simulink model "acquisition"  (R2020a)
settings: Solver=VariableStepAuto  StartTime=0.0  StopTime=simulation_time  RelTol=1e-3
values from neighbouring files (symbols this model uses):
  ca_fft_coef = zeros(37,4096)    [acquisition_hw_init.m]
  ca_fft_width = 14    [acquisition_hw_init.m]
  core_upsample_ratio = 24    [acquisition_hw_init.m]
  correlator_latency = 19    [acquisition_hw_init.m]
  ddc_latency = 5    [acquisition_hw_init.m]
  DDS_signal_width = 12    [acquisition_hw_init.m]
  f_start_phase = core_upsample_ratio*f_start/fs    (= -0.0006103515625)    [acquisition_hw_init.m]
  fd_phase_increment = core_upsample_ratio*(f_dds_change)/fs    (= 2e-05)    [acquisition_hw_init.m]
  fft_length = 4096    [acquisition_hw_init.m]
  fs = core_upsample_ratio*fs_adc    (= 120000000)    [acquisition_hw_init.m]
  ts = 1/fs    [acquisition_debugger_data.m]    (also in acquisition_hw_init.m = 8.33333333333e-09)
  ts_adc = 1/fs_adc    (= 2e-07)    [acquisition_hw_init.m]
libraries: xbsIndex_r4 x325
(part 1 of 2)
settings Model: Creator=NoiseIran  LastModifiedBy=sysgen

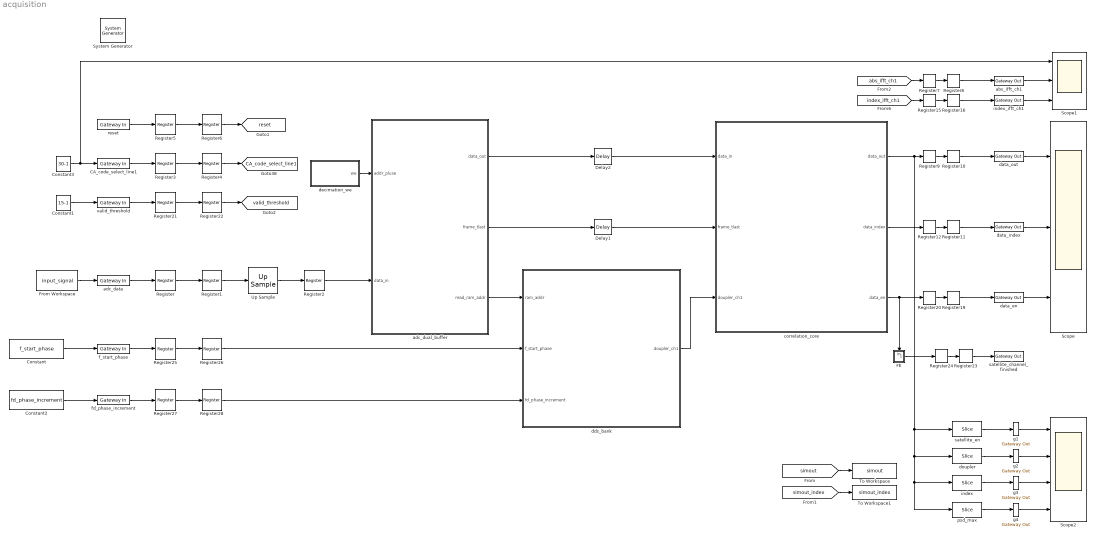
== system acquisition ==
  " System Generator" : xbsIndex_r4/ System Generator  Tag=genX  xilinxfamily=zynq  part=xc7z020  speed=-1  package=clg400  synthesis_tool=Vivado  clock_wrapper=Clock Enables  directory=./netlist  proj_type=Vivado  Synth_file=Vivado Synthesis Defaults  Impl_file=Vivado Implementation Defaults  testbench=off  simulink_period=ts  sysclk_period=ts*1e9  dcm_input_clock_period=10  incr_netlist=off  trim_vbits=Everywhere in SubSystem  dbl_ovrd=According to Block Masks  core_generation=According to Block Masks  run_coregen=off  deprecated_control=off  eval_field=0  block_type=sysgen
  CA_code_select_line1 : xbsIndex_r4/Gateway In  gui_display_data_type=Fixed-point  arith_type=Unsigned  n_bits=6  bin_pt=0  preci_type=Single  exp_width=8  frac_width=24  rows=1  columns=1  quantization="Round  (unbiased: +/- Inf)"  overflow=Saturate  period=ts  UseAsADC=off  ADCChannel='1'  interface=None  automatic_assignment=on  address_offset=hex2dec('00')  intf_name=''  intf_description=''  default_value=0  timing_constraint=None  locs_specified=off  LOCs={}  io_standard={}  inherit_from_input=off  hdl_port=on  dbl_ovrd=off  block_type=gatewayin
  Constant : Constant  Value=f_start_phase
  Constant1 : Constant  Value=15-1
  Constant2 : Constant  Value=fd_phase_increment
  Constant3 : Constant  Value=30-1
  Delay1 : xbsIndex_r4/Delay  rst=off  infoeditControl=Selection of Reset will increase slice count due to use of real FFs and instead of SRLs  en=off  latency=ddc_latency  reg_retiming=off  dbl_ovrd=off  block_type=delay
  Delay2 : xbsIndex_r4/Delay  rst=off  infoeditControl=Selection of Reset will increase slice count due to use of real FFs and instead of SRLs  en=off  latency=ddc_latency  reg_retiming=off  dbl_ovrd=off  block_type=delay
  FE : Subsystem
      settings: PortSchema="{\"entries\":[{\"content\":{\"sides\":[{\"content\":{\"connectorIds\":[]},\"type\":\"ConnectorPlacement.EquallySpacedRectSide\",\"uuid\":\"2043c5b6-9866-4807-b8e4-2bcf4a8da4e0\"},{\"content\":{\"connectorIds\":[\"Out1\"],\"side\":\"RIGHT\"},\"type\":\"ConnectorPlacement.EquallySpacedRectSide\",\"uuid\":\"05fb68c1-bf14-4cfd-8c41-78b1f158a67a\"},{\"content\":{\"connectorIds\":[\"In1\"],\"side\":\"TOP\"},\"type\":\"ConnectorPlacement.EquallySpacedRectSide\",\"uuid\":\"9a584094-bda8-44b5-9f18-145d2f87f2be\"}]},\"type\":\"ConnectorPlacement.EquallySpacedConnector\",\"uuid\":\"61bf9f6d-0cb1-4913-8ccd-914b8e14feb8\"}],\"packageUris\":[\"http://schema.mathworks.com/mf0/Connector/19700101\"],\"version\":\"1.0\"}"
  From Workspace : FromWorkspace  VariableName=input_signal  SampleTime=ts_adc
  Register{,1..4,7..12,15..16,19..28} (23 alike) : xbsIndex_r4/Register  init=0  rst=off  en=off  dbl_ovrd=off  block_type=register
  Register5 : xbsIndex_r4/Register  init=1  rst=off  en=off  dbl_ovrd=off  block_type=register
  Register6 : xbsIndex_r4/Register  init=1  rst=off  en=off  dbl_ovrd=off  block_type=register
  Scope : Scope  NumInputPorts=3
  Scope1 : Scope  NumInputPorts=3
  Scope2 : Scope  NumInputPorts=4
  To Workspace : ToWorkspace  VariableName=simout  SaveFormat=Structure With Time  SampleTime=-1
  To Workspace1 : ToWorkspace  VariableName=simout_index  SaveFormat=Structure With Time  SampleTime=-1
  Up Sample : xbsIndex_r4/Up Sample  sample_ratio=core_upsample_ratio  copy_samples=on  en=off  latency=1  dbl_ovrd=off  block_type=usamp
  abs_ifft_ch1 : xbsIndex_r4/Gateway Out  inherit_from_input=off  hdl_port=on  rows=1  columns=1  UseAsDAC=off  DACChannel='1'  interface=None  automatic_assignment=on  address_offset=hex2dec('00')  intf_name=''  intf_description=''  timing_constraint=None  locs_specified=off  LOCs={}  io_standard={}  block_type=gatewayout
  adc_data : xbsIndex_r4/Gateway In  gui_display_data_type=Fixed-point  arith_type="Signed  (2's comp)"  n_bits=input_signal_width  bin_pt=input_signal_binary_point  preci_type=Single  exp_width=8  frac_width=24  rows=1  columns=1  quantization="Round  (unbiased: +/- Inf)"  overflow=Saturate  period=ts_adc  UseAsADC=off  ADCChannel='1'  interface=None  automatic_assignment=on  address_offset=hex2dec('00')  intf_name=''  intf_description=''  default_value=0  timing_constraint=None  locs_specified=off  LOCs={}  io_standard={}  inherit_from_input=off  hdl_port=on  dbl_ovrd=off  block_type=gatewayin
  adc_dual_buffer : Subsystem
  correlation_core : Subsystem
  data_en : xbsIndex_r4/Gateway Out  inherit_from_input=off  hdl_port=on  rows=1  columns=1  UseAsDAC=off  DACChannel='1'  interface=None  automatic_assignment=on  address_offset=hex2dec('00')  intf_name=''  intf_description=''  timing_constraint=None  locs_specified=off  LOCs={}  io_standard={}  block_type=gatewayout
  data_index : xbsIndex_r4/Gateway Out  inherit_from_input=off  hdl_port=on  rows=1  columns=1  UseAsDAC=off  DACChannel='1'  interface=None  automatic_assignment=on  address_offset=hex2dec('00')  intf_name=''  intf_description=''  timing_constraint=None  locs_specified=off  LOCs={}  io_standard={}  block_type=gatewayout
  data_out : xbsIndex_r4/Gateway Out  inherit_from_input=off  hdl_port=on  rows=1  columns=1  UseAsDAC=off  DACChannel='1'  interface=None  automatic_assignment=on  address_offset=hex2dec('00')  intf_name=''  intf_description=''  timing_constraint=None  locs_specified=off  LOCs={}  io_standard={}  block_type=gatewayout
  dds_bank : Subsystem
  decimation_we : Subsystem
  doupler : xbsIndex_r4/Slice  nbits=24  boolean_output=off  mode=Lower Bit Location + Width  bit1=0  base1=MSB of Input  bit0=20  base0=LSB of Input  dbl_ovrd=off  block_type=slice
  f_start_phase : xbsIndex_r4/Gateway In  gui_display_data_type=Fixed-point  arith_type="Signed  (2's comp)"  n_bits=DDS_phase_width  bin_pt=DDS_phase_width  preci_type=Single  exp_width=8  frac_width=24  rows=1  columns=1  quantization="Round  (unbiased: +/- Inf)"  overflow=Saturate  period=ts  UseAsADC=off  ADCChannel='1'  interface=None  automatic_assignment=on  address_offset=hex2dec('00')  intf_name=''  intf_description=''  default_value=0  timing_constraint=None  locs_specified=off  LOCs={}  io_standard={}  inherit_from_input=off  hdl_port=on  dbl_ovrd=off  block_type=gatewayin
  fd_phase_increment : xbsIndex_r4/Gateway In  gui_display_data_type=Fixed-point  arith_type="Signed  (2's comp)"  n_bits=DDS_phase_width  bin_pt=DDS_phase_width  preci_type=Single  exp_width=8  frac_width=24  rows=1  columns=1  quantization="Round  (unbiased: +/- Inf)"  overflow=Saturate  period=ts  UseAsADC=off  ADCChannel='1'  interface=None  automatic_assignment=on  address_offset=hex2dec('00')  intf_name=''  intf_description=''  default_value=0  timing_constraint=None  locs_specified=off  LOCs={}  io_standard={}  inherit_from_input=off  hdl_port=on  dbl_ovrd=off  block_type=gatewayin
  g{1..4} (4 alike) : xbsIndex_r4/Gateway Out  inherit_from_input=off  hdl_port=off  rows=1  columns=1  UseAsDAC=off  DACChannel='1'  interface=None  automatic_assignment=on  address_offset=hex2dec('00')  intf_name=''  intf_description=''  timing_constraint=None  locs_specified=off  LOCs={}  io_standard={}  block_type=gatewayout
  index : xbsIndex_r4/Slice  nbits=12  boolean_output=off  mode=Lower Bit Location + Width  bit1=0  base1=MSB of Input  bit0=8  base0=LSB of Input  dbl_ovrd=off  block_type=slice
  index_ifft_ch1 : xbsIndex_r4/Gateway Out  inherit_from_input=off  hdl_port=on  rows=1  columns=1  UseAsDAC=off  DACChannel='1'  interface=None  automatic_assignment=on  address_offset=hex2dec('00')  intf_name=''  intf_description=''  timing_constraint=None  locs_specified=off  LOCs={}  io_standard={}  block_type=gatewayout
  psd_max : xbsIndex_r4/Slice  nbits=8  boolean_output=off  mode=Lower Bit Location + Width  bit1=0  base1=MSB of Input  bit0=0  base0=LSB of Input  dbl_ovrd=off  block_type=slice
  reset : xbsIndex_r4/Gateway In  gui_display_data_type=Boolean  arith_type=Boolean  n_bits=4  bin_pt=0  preci_type=Single  exp_width=8  frac_width=24  rows=1  columns=1  quantization="Round  (unbiased: +/- Inf)"  overflow=Saturate  period=ts  UseAsADC=off  ADCChannel='1'  interface=None  automatic_assignment=on  address_offset=hex2dec('00')  intf_name=''  intf_description=''  default_value=0  timing_constraint=None  locs_specified=off  LOCs={}  io_standard={}  inherit_from_input=off  hdl_port=on  dbl_ovrd=off  block_type=gatewayin
  satellite_channel_finished : xbsIndex_r4/Gateway Out  inherit_from_input=off  hdl_port=on  rows=1  columns=1  UseAsDAC=off  DACChannel='1'  interface=None  automatic_assignment=on  address_offset=hex2dec('00')  intf_name=''  intf_description=''  timing_constraint=None  locs_specified=off  LOCs={}  io_standard={}  block_type=gatewayout
  satellite_en : xbsIndex_r4/Slice  nbits=1  boolean_output=on  mode=Lower Bit Location + Width  bit1=0  base1=MSB of Input  bit0=44  base0=LSB of Input  dbl_ovrd=off  block_type=slice
  valid_threshold : xbsIndex_r4/Gateway In  gui_display_data_type=Fixed-point  arith_type="Signed  (2's comp)"  n_bits=abs_adder_width  bin_pt=abs_adder_point  preci_type=Single  exp_width=8  frac_width=24  rows=1  columns=1  quantization="Round  (unbiased: +/- Inf)"  overflow=Saturate  period=ts  UseAsADC=off  ADCChannel='1'  interface=None  automatic_assignment=on  address_offset=hex2dec('00')  intf_name=''  intf_description=''  default_value=0  timing_constraint=None  locs_specified=off  LOCs={}  io_standard={}  inherit_from_input=off  hdl_port=on  dbl_ovrd=off  block_type=gatewayin
  tag scope: CA_code_select_line1=global, reset=global, valid_threshold=global
  wires:
  Register/1 -> Register1/1
  adc_data/1 -> Register/1
  Register1/1 -> Up Sample/1
  Up Sample/1 -> Register2/1
  Register2/1 -> adc_dual_buffer/2(data_in)
  adc_dual_buffer/3(read_ram_addr) -> dds_bank/1(ram_addr)
  From Workspace/1 -> adc_data/1
  adc_dual_buffer/1(data_out) -> Delay2/1
  CA_code_select_line1/1 -> Register3/1
  Register3/1 -> Register4/1
  Register4/1 -> [CA_code_select_line1]
  reset/1 -> Register5/1
  Register5/1 -> Register6/1
  Register6/1 -> [reset]
  decimation_we/1(we) -> adc_dual_buffer/1(addr_pluse)
  Register8/1 -> abs_ifft_ch1/1
  Register7/1 -> Register8/1
  dds_bank/1(doupler_ch1) -> correlation_core/3(doupler_ch1)
  [abs_ifft_ch1] -> Register7/1
  Register16/1 -> index_ifft_ch1/1
  Register15/1 -> Register16/1
  [index_ifft_ch1] -> Register15/1
  correlation_core/1(data_out) -> psd_max/1, index/1, doupler/1, satellite_en/1, Register9/1
  Register9/1 -> Register10/1
  Register11/1 -> data_index/1
  Register12/1 -> Register11/1
  correlation_core/2(data_index) -> Register12/1
  Register20/1 -> Register19/1
  Register19/1 -> data_en/1
  correlation_core/3(data_en) -> FE/1(in), Register20/1
  data_out/1 -> Scope/1
  data_index/1 -> Scope/2
  data_en/1 -> Scope/3
  abs_ifft_ch1/1 -> Scope1/2
  index_ifft_ch1/1 -> Scope1/3
  Register21/1 -> Register22/1
  valid_threshold/1 -> Register21/1
  Register22/1 -> [valid_threshold]
  Constant1/1 -> valid_threshold/1
  Register24/1 -> Register23/1
  Register23/1 -> satellite_channel_finished/1
  FE/1(fe) -> Register24/1
  Register10/1 -> data_out/1
  satellite_en/1 -> g1/1
  doupler/1 -> g2/1
  index/1 -> g3/1
  psd_max/1 -> g4/1
  Constant2/1 -> fd_phase_increment/1
  Constant/1 -> f_start_phase/1
  f_start_phase/1 -> Register25/1
  fd_phase_increment/1 -> Register27/1
  Register25/1 -> Register26/1
  Register26/1 -> dds_bank/2(f_start_phase)
  Register27/1 -> Register28/1
  Register28/1 -> dds_bank/3(fd_phase_increment)
  adc_dual_buffer/2(frame_tlast) -> Delay1/1
  Delay2/1 -> correlation_core/1(data_in)
  Delay1/1 -> correlation_core/2(frame_tlast)
  [simout] -> To Workspace/1
  [simout_index] -> To Workspace1/1
  Constant3/1 -> Scope1/1, CA_code_select_line1/1
  g1/1 -> Scope2/1
  g2/1 -> Scope2/2
  g3/1 -> Scope2/3
  g4/1 -> Scope2/4

== system acquisition/FE ==
  in : Inport
  Delay : xbsIndex_r4/Delay  rst=off  infoeditControl=Selection of Reset will increase slice count due to use of real FFs and instead of SRLs  en=off  latency=1  reg_retiming=off  dbl_ovrd=off  block_type=delay
  Inverter : xbsIndex_r4/Inverter  en=off  latency=0  dbl_ovrd=off  block_type=inv
  Logical : xbsIndex_r4/Logical  logical_function=AND  inputs=2  en=off  latency=0  precision=Full  arith_type=Unsigned  n_bits=16  bin_pt=0  align_bp=on  dbl_ovrd=off  block_type=logical
  fe : Outport
  wires:
  in/1 -> Inverter/1, Delay/1
  Inverter/1 -> Logical/1
  Delay/1 -> Logical/2
  Logical/1 -> fe/1

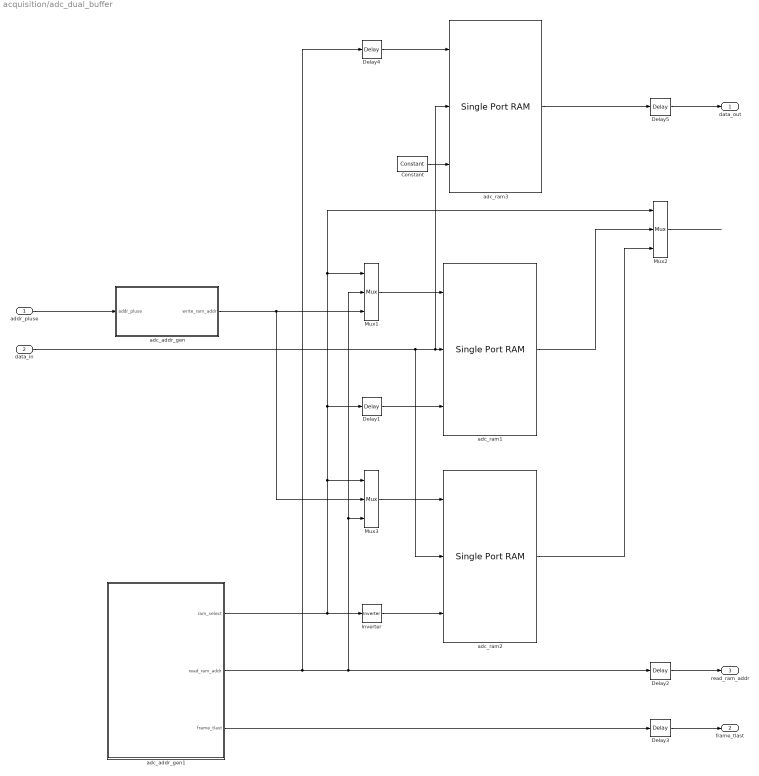
== system acquisition/adc_dual_buffer ==
  addr_pluse : Inport
  data_in : Inport  Port=2
  Constant : xbsIndex_r4/Constant  const=0  gui_display_data_type=Boolean  arith_type=Boolean  n_bits=16  bin_pt=14  preci_type=Single  exp_width=8  frac_width=24  explicit_period=on  period=ts  equ=P=C  opselect=C  inp2=PCIN>>17  opr=+  inp1=P  carry=CIN  dbl_ovrd=off  block_type=constant
  Delay1 : xbsIndex_r4/Delay  rst=off  infoeditControl=Selection of Reset will increase slice count due to use of real FFs and instead of SRLs  en=off  latency=1  reg_retiming=off  dbl_ovrd=off  block_type=delay
  Delay2 : xbsIndex_r4/Delay  rst=off  infoeditControl=Selection of Reset will increase slice count due to use of real FFs and instead of SRLs  en=off  latency=adc_addr_gen_latency  reg_retiming=off  dbl_ovrd=off  block_type=delay
  Delay3 : xbsIndex_r4/Delay  rst=off  infoeditControl=Selection of Reset will increase slice count due to use of real FFs and instead of SRLs  en=off  latency=adc_addr_gen_latency  reg_retiming=off  dbl_ovrd=off  block_type=delay
  Delay4 : xbsIndex_r4/Delay  rst=off  infoeditControl=Selection of Reset will increase slice count due to use of real FFs and instead of SRLs  en=off  latency=1  reg_retiming=off  dbl_ovrd=off  block_type=delay
  Delay5 : xbsIndex_r4/Delay  rst=off  infoeditControl=Selection of Reset will increase slice count due to use of real FFs and instead of SRLs  en=off  latency=1  reg_retiming=off  dbl_ovrd=off  block_type=delay
  Inverter : xbsIndex_r4/Inverter  en=off  latency=1  dbl_ovrd=off  block_type=inv
  Mux1 : xbsIndex_r4/Mux  inputs=2  en=off  latency=1  precision=Full  arith_type=Unsigned  n_bits=16  bin_pt=14  quantization=Truncate  overflow=Wrap  dbl_ovrd=off  block_type=mux
  Mux2 : xbsIndex_r4/Mux  inputs=2  en=off  latency=1  precision=Full  arith_type=Unsigned  n_bits=16  bin_pt=14  quantization=Truncate  overflow=Wrap  dbl_ovrd=off  block_type=mux
  Mux3 : xbsIndex_r4/Mux  inputs=2  en=off  latency=1  precision=Full  arith_type=Unsigned  n_bits=16  bin_pt=14  quantization=Truncate  overflow=Wrap  dbl_ovrd=off  block_type=mux
  adc_addr_gen : Subsystem
  adc_addr_gen1 : Subsystem
  adc_ram1 : xbsIndex_r4/Single Port RAM  depth=fft_length  initVector=adc_ram_init  distributed_mem=Block RAM  write_mode=Read After Write  rst=off  init_reg=0  en=off  optimize_latency=off  latency=1  optimize=Speed  dbl_ovrd=off  simulation_type=fast_sim  block_type=spram
  adc_ram2 : xbsIndex_r4/Single Port RAM  depth=fft_length  initVector=adc_ram_init  distributed_mem=Block RAM  write_mode=Read After Write  rst=off  init_reg=0  en=off  optimize_latency=off  latency=1  optimize=Speed  dbl_ovrd=off  simulation_type=fast_sim  block_type=spram
  adc_ram3 : xbsIndex_r4/Single Port RAM  depth=fft_length  initVector=adc_ram_init  distributed_mem=Block RAM  write_mode=Read After Write  rst=off  init_reg=0  en=off  optimize_latency=off  latency=1  optimize=Speed  dbl_ovrd=off  simulation_type=fast_sim  block_type=spram
  data_out : Outport
  frame_tlast : Outport  Port=2
  read_ram_addr : Outport  Port=3
  wires:
  Mux1/1 -> adc_ram1/1
  Inverter/1 -> adc_ram2/3
  Mux3/1 -> adc_ram2/1
  adc_addr_gen/1(write_ram_addr) -> Mux3/2, Mux1/3
  adc_addr_gen1/1(ram_select) -> Mux2/1, Mux1/1, Delay1/1, Mux3/1, Inverter/1
  adc_ram1/1 -> Mux2/2
  adc_ram2/1 -> Mux2/3
  Delay1/1 -> adc_ram1/3
  addr_pluse/1 -> adc_addr_gen/1(addr_pluse)
  Mux2/1 -> ?
  Delay2/1 -> read_ram_addr/1
  adc_addr_gen1/3(frame_tlast) -> Delay3/1
  Delay3/1 -> frame_tlast/1
  adc_addr_gen1/2(read_ram_addr) -> Delay4/1, Mux1/2, Mux3/3, Delay2/1
  data_in/1 -> adc_ram3/2, adc_ram1/2, adc_ram2/2
  Constant/1 -> adc_ram3/3
  Delay4/1 -> adc_ram3/1
  adc_ram3/1 -> Delay5/1
  Delay5/1 -> data_out/1

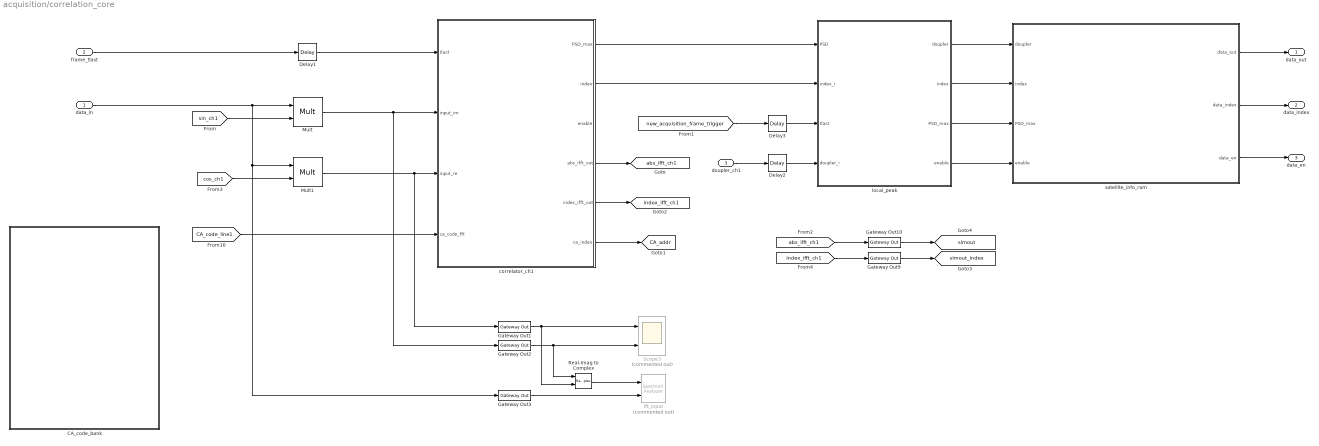
== system acquisition/correlation_core ==
  data_in : Inport
  frame_tlast : Inport  Port=2
  doupler_ch1 : Inport  Port=3
  CA_code_bank : Subsystem
  Delay1 : xbsIndex_r4/Delay  rst=off  infoeditControl=Selection of Reset will increase slice count due to use of real FFs and instead of SRLs  en=off  latency=3  reg_retiming=off  dbl_ovrd=off  block_type=delay
  Delay2 : xbsIndex_r4/Delay  rst=off  infoeditControl=Selection of Reset will increase slice count due to use of real FFs and instead of SRLs  en=off  latency=correlator_latency  reg_retiming=off  dbl_ovrd=off  block_type=delay
  Delay3 : xbsIndex_r4/Delay  rst=off  infoeditControl=Selection of Reset will increase slice count due to use of real FFs and instead of SRLs  en=off  latency=correlator_latency+ddc_latency  reg_retiming=off  dbl_ovrd=off  block_type=delay
  Gateway Out{1..3,9..10} (5 alike) : xbsIndex_r4/Gateway Out  inherit_from_input=off  hdl_port=off  rows=1  columns=1  UseAsDAC=off  DACChannel='1'  interface=None  automatic_assignment=on  address_offset=hex2dec('00')  intf_name=''  intf_description=''  timing_constraint=None  locs_specified=off  LOCs={}  io_standard={}  block_type=gatewayout
  Mult : xbsIndex_r4/Mult  precision=User Defined  arith_type="Signed  (2's comp)"  n_bits=multiplier_width  bin_pt=multiplier_point  quantization="Round  (unbiased: +/- Inf)"  overflow=Saturate  en=off  latency=3  use_behavioral_HDL=off  opt=Speed  use_embedded=on  optimum_pipeline=off  pipeline=on  dbl_ovrd=off  use_rpm=on  placement_style=Triangular  block_type=mult
  Mult1 : xbsIndex_r4/Mult  precision=User Defined  arith_type="Signed  (2's comp)"  n_bits=multiplier_width  bin_pt=multiplier_point  quantization="Round  (unbiased: +/- Inf)"  overflow=Saturate  en=off  latency=3  use_behavioral_HDL=off  opt=Speed  use_embedded=on  optimum_pipeline=off  pipeline=on  dbl_ovrd=off  use_rpm=on  placement_style=Triangular  block_type=mult
  Real-Imag to Complex : RealImagToComplex
  Scope3 : Scope  Commented=on  NumInputPorts=2
  correlator_ch1 : Subsystem
  fft_input : SpectrumAnalyzer  Commented=on  NumInputPorts=2
  local_peak : Subsystem
  satellite_info_ram : Subsystem
  data_out : Outport
  data_index : Outport  Port=2
  data_en : Outport  Port=3
  tag scope: CA_addr=global, abs_ifft_ch1=global, index_ifft_ch1=global, simout=global, simout_index=global
  wires:
  [sin_ch1] -> Mult/2
  [cos_ch1] -> Mult1/2
  frame_tlast/1 -> Delay1/1
  Mult/1 -> Gateway Out2/1, correlator_ch1/2(input_im)
  Mult1/1 -> Gateway Out1/1, correlator_ch1/3(input_re)
  correlator_ch1/6(ca_index) -> [CA_addr]
  [CA_code_line1] -> correlator_ch1/4(ca_code_fft)
  correlator_ch1/4(abs_ifft_out) -> [abs_ifft_ch1]
  correlator_ch1/5(index_ifft_out) -> [index_ifft_ch1]
  doupler_ch1/1 -> Delay2/1
  local_peak/1(doupler) -> satellite_info_ram/1(doupler)
  local_peak/2(index) -> satellite_info_ram/2(index)
  local_peak/3(PSD_max) -> satellite_info_ram/3(PSD_max)
  local_peak/4(enable) -> satellite_info_ram/4(enable)
  satellite_info_ram/1(data_out) -> data_out/1
  satellite_info_ram/2(data_index) -> data_index/1
  satellite_info_ram/3(data_en) -> data_en/1
  Real-Imag to Complex/1 -> fft_input/1
  Gateway Out1/1 -> Real-Imag to Complex/2, Scope3/1
  Gateway Out2/1 -> Real-Imag to Complex/1, Scope3/2
  [new_acquisition_frame_trigger] -> Delay3/1
  correlator_ch1/1(PSD_max) -> local_peak/1(PSD)
  correlator_ch1/2(index) -> local_peak/2(index_i)
  Delay1/1 -> correlator_ch1/1(tlast)
  Delay3/1 -> local_peak/3(tlast)
  Delay2/1 -> local_peak/4(doupler_i)
  data_in/1 -> Gateway Out3/1, Mult1/1, Mult/1
  Gateway Out3/1 -> fft_input/2
  Gateway Out10/1 -> [simout]
  Gateway Out9/1 -> [simout_index]
  [abs_ifft_ch1] -> Gateway Out10/1
  [index_ifft_ch1] -> Gateway Out9/1

== system acquisition/dds_bank ==
  ram_addr : Inport
  f_start_phase : Inport  Port=2
  fd_phase_increment : Inport  Port=3
  Constant1 : xbsIndex_r4/Constant  const=fft_length-1  gui_display_data_type=Fixed-point  arith_type=Unsigned  n_bits=12  bin_pt=0  preci_type=Single  exp_width=8  frac_width=24  explicit_period=off  period=1  equ=P=C  opselect=C  inp2=PCIN>>17  opr=+  inp1=P  carry=CIN  dbl_ovrd=off  block_type=constant
  Constant2 : xbsIndex_r4/Constant  const=5  gui_display_data_type=Fixed-point  arith_type=Unsigned  n_bits=12  bin_pt=0  preci_type=Single  exp_width=8  frac_width=24  explicit_period=on  period=ts  equ=P=C  opselect=C  inp2=PCIN>>17  opr=+  inp1=P  carry=CIN  dbl_ovrd=off  block_type=constant
  Gateway Out3 : xbsIndex_r4/Gateway Out  inherit_from_input=off  hdl_port=off  rows=1  columns=1  UseAsDAC=off  DACChannel='1'  interface=None  automatic_assignment=on  address_offset=hex2dec('00')  intf_name=''  intf_description=''  timing_constraint=None  locs_specified=off  LOCs={}  io_standard={}  block_type=gatewayout
  Gateway Out6 : xbsIndex_r4/Gateway Out  inherit_from_input=off  hdl_port=off  rows=1  columns=1  UseAsDAC=off  DACChannel='1'  interface=None  automatic_assignment=on  address_offset=hex2dec('00')  intf_name=''  intf_description=''  timing_constraint=None  locs_specified=off  LOCs={}  io_standard={}  block_type=gatewayout
  Relational1 : xbsIndex_r4/Relational  mode=a=b  op_type=Bool  en=off  latency=0  dbl_ovrd=off  block_type=relational
  Scope1 : Scope  NumInputPorts=2
  dds_core : Subsystem
  doupler_ch1 : Outport
  tag scope: cos_ch1=global, sin_ch1=global
  wires:
  ram_addr/1 -> ?
  Constant1/1 -> Relational1/2
  f_start_phase/1 -> dds_core/1(f_start_phase)
  Gateway Out6/1 -> Scope1/2
  [cos_ch1] -> Gateway Out6/1
  Gateway Out3/1 -> Scope1/1
  [sin_ch1] -> Gateway Out3/1
  fd_phase_increment/1 -> dds_core/2(fd_phase_increment)
  Relational1/1 -> dds_core/3(phase_increment_update)
  [new_acquisition_frame_trigger] -> dds_core/4(reset_to_f_start)
  dds_core/2(sin) -> [sin_ch1]
  dds_core/1(current_phase) -> doupler_ch1/1
  dds_core/3(cos) -> [cos_ch1]
  Constant2/1 -> Relational1/1

== system acquisition/decimation_we ==
  Constant : xbsIndex_r4/Constant  const=core_upsample_ratio-1  gui_display_data_type=Fixed-point  arith_type=Unsigned  n_bits=8  bin_pt=0  preci_type=Single  exp_width=8  frac_width=24  explicit_period=on  period=ts  equ=P=C  opselect=C  inp2=PCIN>>17  opr=+  inp1=P  carry=CIN  dbl_ovrd=off  block_type=constant
  Counter1 : xbsIndex_r4/Counter  cnt_type=Free Running  cnt_to=Inf  operation=Up  start_count=0  cnt_by_val=1  arith_type=Unsigned  n_bits=8  bin_pt=0  load_pin=off  rst=on  en=off  explicit_period=off  period=1  use_behavioral_HDL=off  implementation=Fabric  dbl_ovrd=off  block_type=counter
  Relational : xbsIndex_r4/Relational  mode=a<=b  op_type=Bool  en=off  latency=0  dbl_ovrd=off  block_type=relational
  we : Outport
  wires:
  Constant/1 -> Relational/1
  Relational/1 -> we/1, Counter1/1
  Counter1/1 -> Relational/2

== system acquisition/adc_dual_buffer/adc_addr_gen ==
  addr_pluse : Inport
  Constant1 : xbsIndex_r4/Constant  const=fft_length-1  gui_display_data_type=Fixed-point  arith_type=Unsigned  n_bits=ceil(log2(fft_length))  bin_pt=0  preci_type=Single  exp_width=8  frac_width=24  explicit_period=off  period=1  equ=P=C  opselect=C  inp2=PCIN>>17  opr=+  inp1=P  carry=CIN  dbl_ovrd=off  block_type=constant
  Counter : xbsIndex_r4/Counter  cnt_type=Free Running  cnt_to=Inf  operation=Up  start_count=0  cnt_by_val=1  arith_type=Unsigned  n_bits=ceil(log2(fft_length))  bin_pt=0  load_pin=off  rst=on  en=on  explicit_period=off  period=1  use_behavioral_HDL=off  implementation=Fabric  dbl_ovrd=off  block_type=counter
  Logical : xbsIndex_r4/Logical  logical_function=AND  inputs=2  en=off  latency=1  precision=Full  arith_type=Unsigned  n_bits=16  bin_pt=0  align_bp=on  dbl_ovrd=off  block_type=logical
  Register : xbsIndex_r4/Register  init=0  rst=on  en=on  dbl_ovrd=off  block_type=register
  Register1 : xbsIndex_r4/Register  init=1  rst=off  en=off  dbl_ovrd=off  block_type=register
  Relational1 : xbsIndex_r4/Relational  mode=a=b  op_type=Bool  en=off  latency=0  dbl_ovrd=off  block_type=relational
  Scope : Scope  Commented=on  NumInputPorts=4
  write_ram_addr : Outport
  wires:
  Constant1/1 -> Relational1/1
  Counter/1 -> Scope/1, write_ram_addr/1, Relational1/2
  Relational1/1 -> Scope/3, Counter/1, Register/2
  Logical/1 -> Scope/4, Counter/2
  [new_acquisition_frame_trigger] -> Register1/1
  addr_pluse/1 -> Logical/2
  Register/1 -> Logical/1
  Register1/1 -> Scope/2, Register/3, Register/1

== system acquisition/adc_dual_buffer/adc_addr_gen1 ==
  Constant1 : xbsIndex_r4/Constant  const=core_upsample_ratio  gui_display_data_type=Fixed-point  arith_type=Unsigned  n_bits=8  bin_pt=0  preci_type=Single  exp_width=8  frac_width=24  explicit_period=off  period=1  equ=P=C  opselect=C  inp2=PCIN>>17  opr=+  inp1=P  carry=CIN  dbl_ovrd=off  block_type=constant
  Constant3 : xbsIndex_r4/Constant  const=fft_length-1  gui_display_data_type=Fixed-point  arith_type=Unsigned  n_bits=ceil(log2(fft_length))  bin_pt=0  preci_type=Single  exp_width=8  frac_width=24  explicit_period=off  period=1  equ=P=C  opselect=C  inp2=PCIN>>17  opr=+  inp1=P  carry=CIN  dbl_ovrd=off  block_type=constant
  Convert : xbsIndex_r4/Convert  gui_display_data_type=Boolean  arith_type=Boolean  n_bits=16  bin_pt=14  float_type=Single  exp_bits=8  fraction_bits=24  quantization=Truncate  overflow=Wrap  en=off  latency=0  pipeline=off  dbl_ovrd=off  block_type=convert
  Counter : xbsIndex_r4/Counter  cnt_type=Free Running  cnt_to=Inf  operation=Up  start_count=0  cnt_by_val=1  arith_type=Unsigned  n_bits=ceil(log2(fft_length))  bin_pt=0  load_pin=off  rst=on  en=on  explicit_period=off  period=1  use_behavioral_HDL=off  implementation=Fabric  dbl_ovrd=off  block_type=counter
  Counter2 : xbsIndex_r4/Counter  cnt_type=Free Running  cnt_to=Inf  operation=Up  start_count=0  cnt_by_val=1  arith_type=Unsigned  n_bits=1  bin_pt=0  load_pin=off  rst=off  en=on  explicit_period=off  period=1  use_behavioral_HDL=off  implementation=Fabric  dbl_ovrd=off  block_type=counter
  Counter3 : xbsIndex_r4/Counter  cnt_type=Free Running  cnt_to=Inf  operation=Up  start_count=0  cnt_by_val=1  arith_type=Unsigned  n_bits=ceil(log2(fft_length))  bin_pt=0  load_pin=off  rst=on  en=off  explicit_period=off  period=1  use_behavioral_HDL=off  implementation=Fabric  dbl_ovrd=off  block_type=counter
  Gateway Out : xbsIndex_r4/Gateway Out  inherit_from_input=off  hdl_port=off  rows=1  columns=1  UseAsDAC=off  DACChannel='1'  interface=None  automatic_assignment=on  address_offset=hex2dec('00')  intf_name=''  intf_description=''  timing_constraint=None  locs_specified=off  LOCs={}  io_standard={}  block_type=gatewayout
  Gateway Out1 : xbsIndex_r4/Gateway Out  inherit_from_input=off  hdl_port=off  rows=1  columns=1  UseAsDAC=off  DACChannel='1'  interface=None  automatic_assignment=on  address_offset=hex2dec('00')  intf_name=''  intf_description=''  timing_constraint=None  locs_specified=off  LOCs={}  io_standard={}  block_type=gatewayout
  Gateway Out2 : xbsIndex_r4/Gateway Out  inherit_from_input=off  hdl_port=off  rows=1  columns=1  UseAsDAC=off  DACChannel='1'  interface=None  automatic_assignment=on  address_offset=hex2dec('00')  intf_name=''  intf_description=''  timing_constraint=None  locs_specified=off  LOCs={}  io_standard={}  block_type=gatewayout
  Logical : xbsIndex_r4/Logical  logical_function=AND  inputs=2  en=off  latency=1  precision=Full  arith_type=Unsigned  n_bits=16  bin_pt=0  align_bp=on  dbl_ovrd=off  block_type=logical
  RE : Subsystem
  Relational1 : xbsIndex_r4/Relational  mode=a<b  op_type=Bool  en=off  latency=0  dbl_ovrd=off  block_type=relational
  Relational2 : xbsIndex_r4/Relational  mode=a<=b  op_type=Bool  en=off  latency=0  dbl_ovrd=off  block_type=relational
  Scope : Scope  NumInputPorts=3
  ram_select : Outport
  read_ram_addr : Outport  Port=2
  frame_tlast : Outport  Port=3
  tag scope: new_acquisition_frame_trigger=global
  wires:
  Constant1/1 -> Relational1/1
  Counter2/1 -> Convert/1
  Counter/1 -> Relational1/2
  Counter3/1 -> Relational2/2, Gateway Out1/1, read_ram_addr/1
  [reset] -> Counter3/1
  Constant3/1 -> Relational2/1
  Logical/1 -> RE/1(In)
  Relational2/1 -> Counter/2, Gateway Out2/1, frame_tlast/1, Logical/2
  Relational1/1 -> Logical/1
  RE/1(Out) -> [new_acquisition_frame_trigger], Counter/1, Counter2/1
  Convert/1 -> Gateway Out/1, ram_select/1
  Gateway Out/1 -> Scope/1
  Gateway Out1/1 -> Scope/2
  Gateway Out2/1 -> Scope/3

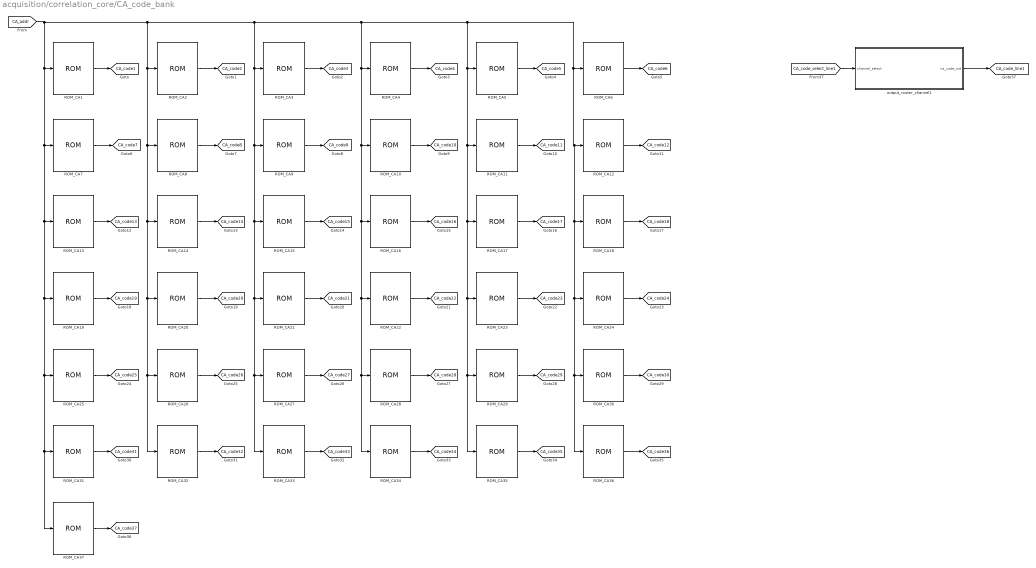
== system acquisition/correlation_core/CA_code_bank ==
  ROM_CA1 : xbsIndex_r4/ROM  depth=4096  initVector=ca_fft_coef(1,:)  distributed_mem=Block RAM  rst=off  init_reg=0  en=off  latency=1  gui_display_data_type=Fixed-point  arith_type=Unsigned  n_bits=2*ca_fft_width  bin_pt=0  preci_type=Single  exp_width=8  frac_width=24  optimize=Area  use_rpm=on  dbl_ovrd=off  simulation_type=fast_sim  block_type=sprom
  ROM_CA10 : xbsIndex_r4/ROM  depth=4096  initVector=ca_fft_coef(10,:)  distributed_mem=Block RAM  rst=off  init_reg=0  en=off  latency=1  gui_display_data_type=Fixed-point  arith_type=Unsigned  n_bits=2*ca_fft_width  bin_pt=0  preci_type=Single  exp_width=8  frac_width=24  optimize=Area  use_rpm=on  dbl_ovrd=off  simulation_type=fast_sim  block_type=sprom
  ROM_CA11 : xbsIndex_r4/ROM  depth=4096  initVector=ca_fft_coef(11,:)  distributed_mem=Block RAM  rst=off  init_reg=0  en=off  latency=1  gui_display_data_type=Fixed-point  arith_type=Unsigned  n_bits=2*ca_fft_width  bin_pt=0  preci_type=Single  exp_width=8  frac_width=24  optimize=Area  use_rpm=on  dbl_ovrd=off  simulation_type=fast_sim  block_type=sprom
  ROM_CA12 : xbsIndex_r4/ROM  depth=4096  initVector=ca_fft_coef(12,:)  distributed_mem=Block RAM  rst=off  init_reg=0  en=off  latency=1  gui_display_data_type=Fixed-point  arith_type=Unsigned  n_bits=2*ca_fft_width  bin_pt=0  preci_type=Single  exp_width=8  frac_width=24  optimize=Area  use_rpm=on  dbl_ovrd=off  simulation_type=fast_sim  block_type=sprom
  ROM_CA13 : xbsIndex_r4/ROM  depth=4096  initVector=ca_fft_coef(13,:)  distributed_mem=Block RAM  rst=off  init_reg=0  en=off  latency=1  gui_display_data_type=Fixed-point  arith_type=Unsigned  n_bits=2*ca_fft_width  bin_pt=0  preci_type=Single  exp_width=8  frac_width=24  optimize=Area  use_rpm=on  dbl_ovrd=off  simulation_type=fast_sim  block_type=sprom
  ROM_CA14 : xbsIndex_r4/ROM  depth=4096  initVector=ca_fft_coef(14,:)  distributed_mem=Block RAM  rst=off  init_reg=0  en=off  latency=1  gui_display_data_type=Fixed-point  arith_type=Unsigned  n_bits=2*ca_fft_width  bin_pt=0  preci_type=Single  exp_width=8  frac_width=24  optimize=Area  use_rpm=on  dbl_ovrd=off  simulation_type=fast_sim  block_type=sprom
  ROM_CA15 : xbsIndex_r4/ROM  depth=4096  initVector=ca_fft_coef(15,:)  distributed_mem=Block RAM  rst=off  init_reg=0  en=off  latency=1  gui_display_data_type=Fixed-point  arith_type=Unsigned  n_bits=2*ca_fft_width  bin_pt=0  preci_type=Single  exp_width=8  frac_width=24  optimize=Area  use_rpm=on  dbl_ovrd=off  simulation_type=fast_sim  block_type=sprom
  ROM_CA16 : xbsIndex_r4/ROM  depth=4096  initVector=ca_fft_coef(16,:)  distributed_mem=Block RAM  rst=off  init_reg=0  en=off  latency=1  gui_display_data_type=Fixed-point  arith_type=Unsigned  n_bits=2*ca_fft_width  bin_pt=0  preci_type=Single  exp_width=8  frac_width=24  optimize=Area  use_rpm=on  dbl_ovrd=off  simulation_type=fast_sim  block_type=sprom
  ROM_CA17 : xbsIndex_r4/ROM  depth=4096  initVector=ca_fft_coef(17,:)  distributed_mem=Block RAM  rst=off  init_reg=0  en=off  latency=1  gui_display_data_type=Fixed-point  arith_type=Unsigned  n_bits=2*ca_fft_width  bin_pt=0  preci_type=Single  exp_width=8  frac_width=24  optimize=Area  use_rpm=on  dbl_ovrd=off  simulation_type=fast_sim  block_type=sprom
  ROM_CA18 : xbsIndex_r4/ROM  depth=4096  initVector=ca_fft_coef(18,:)  distributed_mem=Block RAM  rst=off  init_reg=0  en=off  latency=1  gui_display_data_type=Fixed-point  arith_type=Unsigned  n_bits=2*ca_fft_width  bin_pt=0  preci_type=Single  exp_width=8  frac_width=24  optimize=Area  use_rpm=on  dbl_ovrd=off  simulation_type=fast_sim  block_type=sprom
  ROM_CA19 : xbsIndex_r4/ROM  depth=4096  initVector=ca_fft_coef(19,:)  distributed_mem=Block RAM  rst=off  init_reg=0  en=off  latency=1  gui_display_data_type=Fixed-point  arith_type=Unsigned  n_bits=2*ca_fft_width  bin_pt=0  preci_type=Single  exp_width=8  frac_width=24  optimize=Area  use_rpm=on  dbl_ovrd=off  simulation_type=fast_sim  block_type=sprom
  ROM_CA2 : xbsIndex_r4/ROM  depth=4096  initVector=ca_fft_coef(2,:)  distributed_mem=Block RAM  rst=off  init_reg=0  en=off  latency=1  gui_display_data_type=Fixed-point  arith_type=Unsigned  n_bits=2*ca_fft_width  bin_pt=0  preci_type=Single  exp_width=8  frac_width=24  optimize=Area  use_rpm=on  dbl_ovrd=off  simulation_type=fast_sim  block_type=sprom
  ROM_CA20 : xbsIndex_r4/ROM  depth=4096  initVector=ca_fft_coef(20,:)  distributed_mem=Block RAM  rst=off  init_reg=0  en=off  latency=1  gui_display_data_type=Fixed-point  arith_type=Unsigned  n_bits=2*ca_fft_width  bin_pt=0  preci_type=Single  exp_width=8  frac_width=24  optimize=Area  use_rpm=on  dbl_ovrd=off  simulation_type=fast_sim  block_type=sprom
  ROM_CA21 : xbsIndex_r4/ROM  depth=4096  initVector=ca_fft_coef(21,:)  distributed_mem=Block RAM  rst=off  init_reg=0  en=off  latency=1  gui_display_data_type=Fixed-point  arith_type=Unsigned  n_bits=2*ca_fft_width  bin_pt=0  preci_type=Single  exp_width=8  frac_width=24  optimize=Area  use_rpm=on  dbl_ovrd=off  simulation_type=fast_sim  block_type=sprom
  ROM_CA22 : xbsIndex_r4/ROM  depth=4096  initVector=ca_fft_coef(22,:)  distributed_mem=Block RAM  rst=off  init_reg=0  en=off  latency=1  gui_display_data_type=Fixed-point  arith_type=Unsigned  n_bits=2*ca_fft_width  bin_pt=0  preci_type=Single  exp_width=8  frac_width=24  optimize=Area  use_rpm=on  dbl_ovrd=off  simulation_type=fast_sim  block_type=sprom
  ROM_CA23 : xbsIndex_r4/ROM  depth=4096  initVector=ca_fft_coef(23,:)  distributed_mem=Block RAM  rst=off  init_reg=0  en=off  latency=1  gui_display_data_type=Fixed-point  arith_type=Unsigned  n_bits=2*ca_fft_width  bin_pt=0  preci_type=Single  exp_width=8  frac_width=24  optimize=Area  use_rpm=on  dbl_ovrd=off  simulation_type=fast_sim  block_type=sprom
  ROM_CA24 : xbsIndex_r4/ROM  depth=4096  initVector=ca_fft_coef(24,:)  distributed_mem=Block RAM  rst=off  init_reg=0  en=off  latency=1  gui_display_data_type=Fixed-point  arith_type=Unsigned  n_bits=2*ca_fft_width  bin_pt=0  preci_type=Single  exp_width=8  frac_width=24  optimize=Area  use_rpm=on  dbl_ovrd=off  simulation_type=fast_sim  block_type=sprom
  ROM_CA25 : xbsIndex_r4/ROM  depth=4096  initVector=ca_fft_coef(25,:)  distributed_mem=Block RAM  rst=off  init_reg=0  en=off  latency=1  gui_display_data_type=Fixed-point  arith_type=Unsigned  n_bits=2*ca_fft_width  bin_pt=0  preci_type=Single  exp_width=8  frac_width=24  optimize=Area  use_rpm=on  dbl_ovrd=off  simulation_type=fast_sim  block_type=sprom
  ROM_CA26 : xbsIndex_r4/ROM  depth=4096  initVector=ca_fft_coef(26,:)  distributed_mem=Block RAM  rst=off  init_reg=0  en=off  latency=1  gui_display_data_type=Fixed-point  arith_type=Unsigned  n_bits=2*ca_fft_width  bin_pt=0  preci_type=Single  exp_width=8  frac_width=24  optimize=Area  use_rpm=on  dbl_ovrd=off  simulation_type=fast_sim  block_type=sprom
  ROM_CA27 : xbsIndex_r4/ROM  depth=4096  initVector=ca_fft_coef(27,:)  distributed_mem=Block RAM  rst=off  init_reg=0  en=off  latency=1  gui_display_data_type=Fixed-point  arith_type=Unsigned  n_bits=2*ca_fft_width  bin_pt=0  preci_type=Single  exp_width=8  frac_width=24  optimize=Area  use_rpm=on  dbl_ovrd=off  simulation_type=fast_sim  block_type=sprom
  ROM_CA28 : xbsIndex_r4/ROM  depth=4096  initVector=ca_fft_coef(28,:)  distributed_mem=Block RAM  rst=off  init_reg=0  en=off  latency=1  gui_display_data_type=Fixed-point  arith_type=Unsigned  n_bits=2*ca_fft_width  bin_pt=0  preci_type=Single  exp_width=8  frac_width=24  optimize=Area  use_rpm=on  dbl_ovrd=off  simulation_type=fast_sim  block_type=sprom
  ROM_CA29 : xbsIndex_r4/ROM  depth=4096  initVector=ca_fft_coef(29,:)  distributed_mem=Block RAM  rst=off  init_reg=0  en=off  latency=1  gui_display_data_type=Fixed-point  arith_type=Unsigned  n_bits=2*ca_fft_width  bin_pt=0  preci_type=Single  exp_width=8  frac_width=24  optimize=Area  use_rpm=on  dbl_ovrd=off  simulation_type=fast_sim  block_type=sprom
  ROM_CA3 : xbsIndex_r4/ROM  depth=4096  initVector=ca_fft_coef(3,:)  distributed_mem=Block RAM  rst=off  init_reg=0  en=off  latency=1  gui_display_data_type=Fixed-point  arith_type=Unsigned  n_bits=2*ca_fft_width  bin_pt=0  preci_type=Single  exp_width=8  frac_width=24  optimize=Area  use_rpm=on  dbl_ovrd=off  simulation_type=fast_sim  block_type=sprom
  ROM_CA30 : xbsIndex_r4/ROM  depth=4096  initVector=ca_fft_coef(30,:)  distributed_mem=Block RAM  rst=off  init_reg=0  en=off  latency=1  gui_display_data_type=Fixed-point  arith_type=Unsigned  n_bits=2*ca_fft_width  bin_pt=0  preci_type=Single  exp_width=8  frac_width=24  optimize=Area  use_rpm=on  dbl_ovrd=off  simulation_type=fast_sim  block_type=sprom
  ROM_CA31 : xbsIndex_r4/ROM  depth=4096  initVector=ca_fft_coef(31,:)  distributed_mem=Block RAM  rst=off  init_reg=0  en=off  latency=1  gui_display_data_type=Fixed-point  arith_type=Unsigned  n_bits=2*ca_fft_width  bin_pt=0  preci_type=Single  exp_width=8  frac_width=24  optimize=Area  use_rpm=on  dbl_ovrd=off  simulation_type=fast_sim  block_type=sprom
  ROM_CA32 : xbsIndex_r4/ROM  depth=4096  initVector=ca_fft_coef(32,:)  distributed_mem=Block RAM  rst=off  init_reg=0  en=off  latency=1  gui_display_data_type=Fixed-point  arith_type=Unsigned  n_bits=2*ca_fft_width  bin_pt=0  preci_type=Single  exp_width=8  frac_width=24  optimize=Area  use_rpm=on  dbl_ovrd=off  simulation_type=fast_sim  block_type=sprom
  ROM_CA33 : xbsIndex_r4/ROM  depth=4096  initVector=ca_fft_coef(33,:)  distributed_mem=Block RAM  rst=off  init_reg=0  en=off  latency=1  gui_display_data_type=Fixed-point  arith_type=Unsigned  n_bits=2*ca_fft_width  bin_pt=0  preci_type=Single  exp_width=8  frac_width=24  optimize=Area  use_rpm=on  dbl_ovrd=off  simulation_type=fast_sim  block_type=sprom
  ROM_CA34 : xbsIndex_r4/ROM  depth=4096  initVector=ca_fft_coef(34,:)  distributed_mem=Block RAM  rst=off  init_reg=0  en=off  latency=1  gui_display_data_type=Fixed-point  arith_type=Unsigned  n_bits=2*ca_fft_width  bin_pt=0  preci_type=Single  exp_width=8  frac_width=24  optimize=Area  use_rpm=on  dbl_ovrd=off  simulation_type=fast_sim  block_type=sprom
  ROM_CA35 : xbsIndex_r4/ROM  depth=4096  initVector=ca_fft_coef(35,:)  distributed_mem=Block RAM  rst=off  init_reg=0  en=off  latency=1  gui_display_data_type=Fixed-point  arith_type=Unsigned  n_bits=2*ca_fft_width  bin_pt=0  preci_type=Single  exp_width=8  frac_width=24  optimize=Area  use_rpm=on  dbl_ovrd=off  simulation_type=fast_sim  block_type=sprom
  ROM_CA36 : xbsIndex_r4/ROM  depth=4096  initVector=ca_fft_coef(36,:)  distributed_mem=Block RAM  rst=off  init_reg=0  en=off  latency=1  gui_display_data_type=Fixed-point  arith_type=Unsigned  n_bits=2*ca_fft_width  bin_pt=0  preci_type=Single  exp_width=8  frac_width=24  optimize=Area  use_rpm=on  dbl_ovrd=off  simulation_type=fast_sim  block_type=sprom
  ROM_CA37 : xbsIndex_r4/ROM  depth=4096  initVector=ca_fft_coef(37,:)  distributed_mem=Block RAM  rst=off  init_reg=0  en=off  latency=1  gui_display_data_type=Fixed-point  arith_type=Unsigned  n_bits=2*ca_fft_width  bin_pt=0  preci_type=Single  exp_width=8  frac_width=24  optimize=Area  use_rpm=on  dbl_ovrd=off  simulation_type=fast_sim  block_type=sprom
  ROM_CA4 : xbsIndex_r4/ROM  depth=4096  initVector=ca_fft_coef(4,:)  distributed_mem=Block RAM  rst=off  init_reg=0  en=off  latency=1  gui_display_data_type=Fixed-point  arith_type=Unsigned  n_bits=2*ca_fft_width  bin_pt=0  preci_type=Single  exp_width=8  frac_width=24  optimize=Area  use_rpm=on  dbl_ovrd=off  simulation_type=fast_sim  block_type=sprom
  ROM_CA5 : xbsIndex_r4/ROM  depth=4096  initVector=ca_fft_coef(5,:)  distributed_mem=Block RAM  rst=off  init_reg=0  en=off  latency=1  gui_display_data_type=Fixed-point  arith_type=Unsigned  n_bits=2*ca_fft_width  bin_pt=0  preci_type=Single  exp_width=8  frac_width=24  optimize=Area  use_rpm=on  dbl_ovrd=off  simulation_type=fast_sim  block_type=sprom
  ROM_CA6 : xbsIndex_r4/ROM  depth=4096  initVector=ca_fft_coef(6,:)  distributed_mem=Block RAM  rst=off  init_reg=0  en=off  latency=1  gui_display_data_type=Fixed-point  arith_type=Unsigned  n_bits=2*ca_fft_width  bin_pt=0  preci_type=Single  exp_width=8  frac_width=24  optimize=Area  use_rpm=on  dbl_ovrd=off  simulation_type=fast_sim  block_type=sprom
  ROM_CA7 : xbsIndex_r4/ROM  depth=4096  initVector=ca_fft_coef(7,:)  distributed_mem=Block RAM  rst=off  init_reg=0  en=off  latency=1  gui_display_data_type=Fixed-point  arith_type=Unsigned  n_bits=2*ca_fft_width  bin_pt=0  preci_type=Single  exp_width=8  frac_width=24  optimize=Area  use_rpm=on  dbl_ovrd=off  simulation_type=fast_sim  block_type=sprom
  ROM_CA8 : xbsIndex_r4/ROM  depth=4096  initVector=ca_fft_coef(8,:)  distributed_mem=Block RAM  rst=off  init_reg=0  en=off  latency=1  gui_display_data_type=Fixed-point  arith_type=Unsigned  n_bits=2*ca_fft_width  bin_pt=0  preci_type=Single  exp_width=8  frac_width=24  optimize=Area  use_rpm=on  dbl_ovrd=off  simulation_type=fast_sim  block_type=sprom
  ROM_CA9 : xbsIndex_r4/ROM  depth=4096  initVector=ca_fft_coef(9,:)  distributed_mem=Block RAM  rst=off  init_reg=0  en=off  latency=1  gui_display_data_type=Fixed-point  arith_type=Unsigned  n_bits=2*ca_fft_width  bin_pt=0  preci_type=Single  exp_width=8  frac_width=24  optimize=Area  use_rpm=on  dbl_ovrd=off  simulation_type=fast_sim  block_type=sprom
  output_router_channel1 : Subsystem
  tag scope: CA_code10=global, CA_code11=global, CA_code12=global, CA_code13=global, CA_code14=global, CA_code15=global, CA_code16=global, CA_code17=global, CA_code18=global, CA_code19=global, CA_code1=global, CA_code20=global, CA_code21=global, CA_code22=global, CA_code23=global, CA_code24=global, CA_code25=global, CA_code26=global, CA_code27=global, CA_code28=global, CA_code29=global, CA_code2=global, CA_code30=global, CA_code31=global, CA_code32=global, CA_code33=global, CA_code34=global, CA_code35=global, CA_code36=global, CA_code37=global, CA_code3=global, CA_code4=global, CA_code5=global, CA_code6=global, CA_code7=global, CA_code8=global, CA_code9=global, CA_code_line1=global
  wires:
  ROM_CA1/1 -> [CA_code1]
  ROM_CA2/1 -> [CA_code2]
  ROM_CA3/1 -> [CA_code3]
  ROM_CA4/1 -> [CA_code4]
  ROM_CA5/1 -> [CA_code5]
  ROM_CA6/1 -> [CA_code6]
  ROM_CA7/1 -> [CA_code7]
  ROM_CA8/1 -> [CA_code8]
  ROM_CA9/1 -> [CA_code9]
  ROM_CA10/1 -> [CA_code10]
  ROM_CA11/1 -> [CA_code11]
  ROM_CA12/1 -> [CA_code12]
  ROM_CA13/1 -> [CA_code13]
  ROM_CA14/1 -> [CA_code14]
  ROM_CA15/1 -> [CA_code15]
  ROM_CA16/1 -> [CA_code16]
  ROM_CA17/1 -> [CA_code17]
  ROM_CA18/1 -> [CA_code18]
  ROM_CA19/1 -> [CA_code19]
  [CA_addr] -> ROM_CA7/1, ROM_CA13/1, ROM_CA19/1, ROM_CA25/1, ROM_CA37/1, ROM_CA31/1, ROM_CA1/1, ROM_CA4/1, ROM_CA10/1, ROM_CA16/1, ROM_CA22/1, ROM_CA34/1, ROM_CA28/1, ROM_CA6/1, ROM_CA12/1, ROM_CA18/1, ROM_CA24/1, ROM_CA36/1, ROM_CA30/1, ROM_CA5/1, ROM_CA11/1, ROM_CA17/1, ROM_CA23/1, ROM_CA35/1, ROM_CA29/1, ROM_CA3/1, ROM_CA9/1, ROM_CA15/1, ROM_CA21/1, ROM_CA33/1, ROM_CA27/1, ROM_CA2/1, ROM_CA8/1, ROM_CA14/1, ROM_CA20/1, ROM_CA32/1, ROM_CA26/1
  ROM_CA20/1 -> [CA_code20]
  ROM_CA21/1 -> [CA_code21]
  ROM_CA22/1 -> [CA_code22]
  ROM_CA23/1 -> [CA_code23]
  ROM_CA24/1 -> [CA_code24]
  ROM_CA25/1 -> [CA_code25]
  ROM_CA26/1 -> [CA_code26]
  ROM_CA27/1 -> [CA_code27]
  ROM_CA28/1 -> [CA_code28]
  ROM_CA29/1 -> [CA_code29]
  ROM_CA30/1 -> [CA_code30]
  ROM_CA31/1 -> [CA_code31]
  ROM_CA32/1 -> [CA_code32]
  ROM_CA33/1 -> [CA_code33]
  ROM_CA34/1 -> [CA_code34]
  ROM_CA35/1 -> [CA_code35]
  ROM_CA36/1 -> [CA_code36]
  ROM_CA37/1 -> [CA_code37]
  output_router_channel1/1(ca_code_out) -> [CA_code_line1]
  [CA_code_select_line1] -> output_router_channel1/1(channel_select)

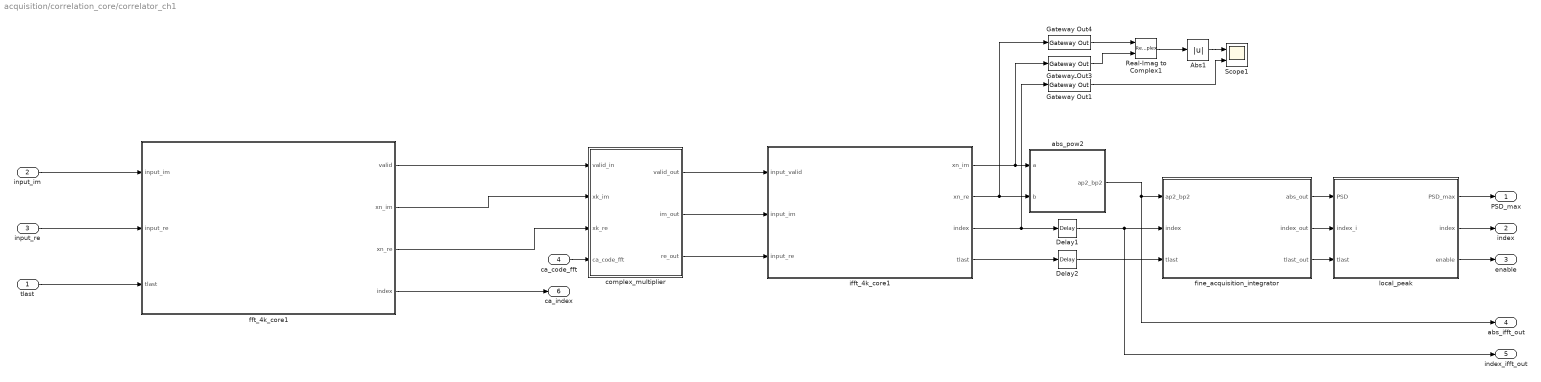
== system acquisition/correlation_core/correlator_ch1 ==
  tlast : Inport
  input_im : Inport  Port=2
  input_re : Inport  Port=3
  ca_code_fft : Inport  Port=4
  Abs1 : Abs
  Delay1 : xbsIndex_r4/Delay  rst=off  infoeditControl=Selection of Reset will increase slice count due to use of real FFs and instead of SRLs  en=off  latency=4  reg_retiming=off  dbl_ovrd=off  block_type=delay
  Delay2 : xbsIndex_r4/Delay  rst=off  infoeditControl=Selection of Reset will increase slice count due to use of real FFs and instead of SRLs  en=off  latency=4  reg_retiming=off  dbl_ovrd=off  block_type=delay
  Gateway Out1 : xbsIndex_r4/Gateway Out  inherit_from_input=off  hdl_port=off  rows=1  columns=1  UseAsDAC=off  DACChannel='1'  interface=None  automatic_assignment=on  address_offset=hex2dec('00')  intf_name=''  intf_description=''  timing_constraint=None  locs_specified=off  LOCs={}  io_standard={}  block_type=gatewayout
  Gateway Out3 : xbsIndex_r4/Gateway Out  inherit_from_input=off  hdl_port=off  rows=1  columns=1  UseAsDAC=off  DACChannel='1'  interface=None  automatic_assignment=on  address_offset=hex2dec('00')  intf_name=''  intf_description=''  timing_constraint=None  locs_specified=off  LOCs={}  io_standard={}  block_type=gatewayout
  Gateway Out4 : xbsIndex_r4/Gateway Out  inherit_from_input=off  hdl_port=off  rows=1  columns=1  UseAsDAC=off  DACChannel='1'  interface=None  automatic_assignment=on  address_offset=hex2dec('00')  intf_name=''  intf_description=''  timing_constraint=None  locs_specified=off  LOCs={}  io_standard={}  block_type=gatewayout
  Real-Imag to Complex1 : RealImagToComplex
  Scope1 : Scope  NumInputPorts=2
  abs_pow2 : Subsystem
  complex_multiplier : Subsystem
  fft_4k_core1 : Subsystem
  fine_acquisition_integrator : Subsystem
  ifft_4k_core1 : Subsystem
  local_peak : Subsystem
  PSD_max : Outport
  index : Outport  Port=2
  enable : Outport  Port=3
  abs_ifft_out : Outport  Port=4
  index_ifft_out : Outport  Port=5
  ca_index : Outport  Port=6
  wires:
  ifft_4k_core1/3(index) -> Gateway Out1/1, Delay1/1
  abs_pow2/1(ap2_bp2) -> fine_acquisition_integrator/1(ap2_bp2), abs_ifft_out/1
  Delay1/1 -> fine_acquisition_integrator/2(index), index_ifft_out/1
  complex_multiplier/1(valid_out) -> ifft_4k_core1/1(input_valid)
  input_im/1 -> fft_4k_core1/1(input_im)
  ifft_4k_core1/1(xn_im) -> Gateway Out3/1, abs_pow2/1(a)
  ifft_4k_core1/2(xn_re) -> Gateway Out4/1, abs_pow2/2(b)
  fft_4k_core1/1(valid) -> complex_multiplier/1(valid_in)
  tlast/1 -> fft_4k_core1/3(tlast)
  ifft_4k_core1/4(tlast) -> Delay2/1
  fft_4k_core1/3(xn_re) -> complex_multiplier/3(xk_re)
  input_re/1 -> fft_4k_core1/2(input_re)
  local_peak/2(index) -> index/1
  local_peak/1(PSD_max) -> PSD_max/1
  local_peak/3(enable) -> enable/1
  ca_code_fft/1 -> complex_multiplier/4(ca_code_fft)
  fft_4k_core1/4(index) -> ca_index/1
  Delay2/1 -> fine_acquisition_integrator/3(tlast)
  fine_acquisition_integrator/1(abs_out) -> local_peak/1(PSD)
  fine_acquisition_integrator/2(index_out) -> local_peak/2(index_i)
  fine_acquisition_integrator/3(tlast_out) -> local_peak/3(tlast)
  Abs1/1 -> Scope1/1
  Real-Imag to Complex1/1 -> Abs1/1
  Gateway Out4/1 -> Real-Imag to Complex1/1
  Gateway Out3/1 -> Real-Imag to Complex1/2
  fft_4k_core1/2(xn_im) -> complex_multiplier/2(xk_im)
  complex_multiplier/2(im_out) -> ifft_4k_core1/2(input_im)
  complex_multiplier/3(re_out) -> ifft_4k_core1/3(input_re)
  Gateway Out1/1 -> Scope1/2
